simulink model "DTC_section2016b"  (R2016b)
settings: Solver=ode23tb  StartTime=0.0  StopTime=0.4  FixedStep=1e-5  MaxStep=2e-6  RelTol=1e-4  EnableMultiTasking=on
InitFcn:
  | R=1.2;
  | pn=4;
  | Ls=0.0085;
  | phaif=0.175;
libraries: powerlib x5, powerlib_meascontrol x1, simulink x1
settings Model: Creator=miracle  LastModifiedBy=Lei
settings SolverCC: ZeroCrossAlgorithm=Adaptive
settings DataIOCC: SaveFormat=StructureWithTime
settings OptimizationCC: LifeSpan=inf
settings DebuggingCC: SFUnexpectedBacktrackingDiag=warning  SFNoUnconditionalDefaultTransitionDiag=warning  SFExecutionAtInitializationDiag=none
settings HardwareCC: ProdBitPerSizeT=32  ProdBitPerPtrDiffT=32  ProdWordSize=32  ProdHWDeviceType=Specified
settings GRTTargetCC: TargetLangStandard=C89/C90 (ANSI)  GeneratePreprocessorConditionals=Disable all
settings ConfigComp: CovMetricSettings=dw  CovHtmlReporting=on  CovSaveCumulativeToWorkspaceVar=on  CovSaveSingleToWorkspaceVar=on  CovExternalEMLEnable=off
settings SimscapeCC: SimscapeNormalizeSystem=off

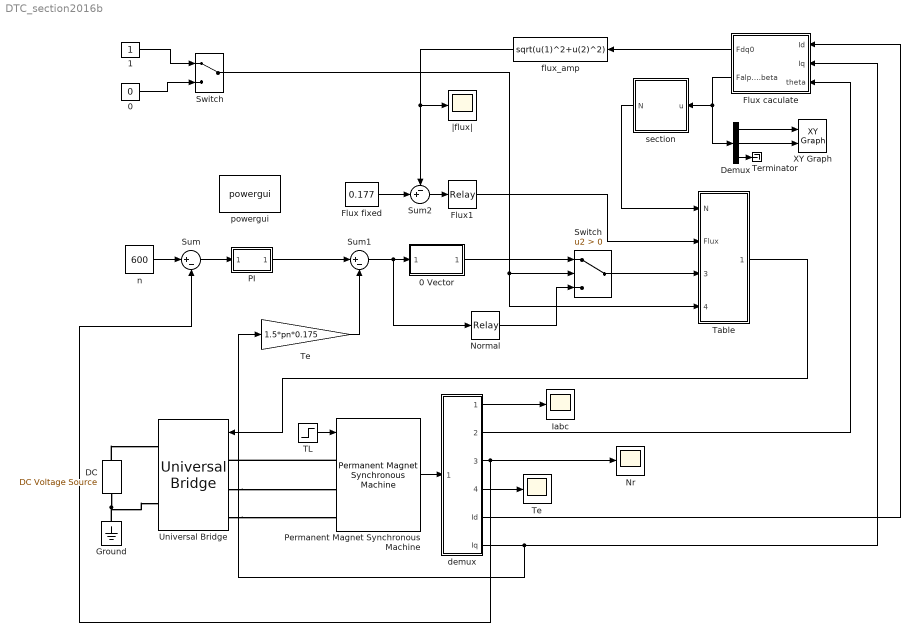
== system DTC_section2016b ==
  " Switch" : ManualSwitch
  0 : Constant  Value=0
  0 Vector : Subsystem
  1 : Constant
  DC : powerlib/Electrical Sources/DC Voltage Source  Amplitude=311  Measurements=None
  Demux : Demux  Outputs=3
  Flux caculate : Subsystem
  Flux fixed : Constant  Value=0.177
  Flux1 : Relay  OnSwitchValue=0.002  OffSwitchValue=-0.002
  Ground : powerlib/Elements/Ground  LConnTagsString=a
  Iabc : Scope
  Normal : Relay  OnSwitchValue=0.15  OffSwitchValue=-0.15
  Nr : Scope
  PI : Subsystem
  Permanent Magnet Synchronous Machine : powerlib/Machines/Permanent Magnet Synchronous Machine  NbPhases=3  FluxDistribution=Sinusoidal  RotorType=Salient-pole  MechanicalLoad=Torque Tm  PresetModel=No  ShowDetailedParameters=on  MeasurementBus=off  Resistance=R  Inductance=8.5e-3  dqInductances=[8.5e-3,8.5e-3]  La=Ls  MachineConstant=Flux linkage established by magnets (V.s)  Flux=phaif  VoltageCst=126.966  TorqueCst=1.05  Flat=120  Mechanical=[0.0008 0.0008 pn 0]  PolePairs=4  InitialConditions=[0,0, 0,0]  InitialConditions5ph=[0 0 0 0 0 0]  TsPowergui=0  TsBlock=-1  RefAngle=Aligned with phase A axis (original Park)
  Sum : Sum  Inputs=|+-
  Sum1 : Sum  Inputs=|+-
  Sum2 : Sum  Inputs=-+|
  Switch : Switch  Criteria=u2 > Threshold
  TL : Step  Time=0.2  After=1.5  SampleTime=0
  Table : Subsystem
  Te : Gain  Gain=1.5*pn*0.175
  "Te " : Scope
  Terminator : Terminator
  Universal Bridge : powerlib/Power Electronics/Universal Bridge  Arms=3  SnubberResistance=1e5  SnubberCapacitance=inf  Device=IGBT / Diodes  Ron=1e-3  Lon=0  ForwardVoltages="[  0  0  ]"  ForwardVoltage=0  GTOparameters=[ 10e-6 , 20e-6 ]  IGBTparameters=[ 1e-6 , 2e-6 ]  Measurements=None  Measurements_2=None  converterType=Rectifier
  XY Graph : simulink/Sinks/XY Graph  xmin=-0.3  xmax=0.3  ymin=-0.3  ymax=0.3  st=-1
  demux : Subsystem
  flux_amp : Fcn  Expr=sqrt(u(1)^2+u(2)^2)
  n : Constant  Value=600
  powergui : powerlib/powergui  Priority=1  SimulationMode=Continuous  SampleTime=50e-6  frequency=60  Iterations=50  frequencyindice=0  Pbase=100e6  ErrMax=1e-4  UnitsV=kV  UnitsW=MW  buscounter=0  FunctionMessages=off  echomessages=off  EnableUseOfTLC=off  CurrentSourceSwitches=on  DisableSnubberDevices=off  DisableRonSwitches=off  DisableVfSwitches=off  DisplayEquations=off  SolverType=Tustin/Backward Euler (TBE)  Interpol=off  ExternalGateDelay=off  methode=off  Ts=10  x0status=blocks  SPID=off  SwTol=0  HookPort=off  RestoreLinks=warning  ResistiveCurrentMeasurement=off  Frange=[0:2:500]  Ylog=off  Xlog=on  ShowGrid=off  save=off  variable=ZData  structure=0  ZoomFFT=off  StartTime=0.0  cycles=1  DisplayStyle=1  fundamental=60  FreqAxis=off  MaxFrequency=1000  frequencyindicesteady=1  RmsSteady=1  display=off
  section : MATLAB Function  TreatAsAtomicUnit=on
  |flux| : Scope
  wires:
  n/1 -> Sum/1
  Sum1/1 -> 0 Vector/1(deltaT), Normal/1
  PI/1(Out1) -> Sum1/1
  TL/1 -> Permanent Magnet Synchronous Machine/1
  Sum2/1 -> Flux1/1
  flux_amp/1 -> Sum2/1, |flux|/1
  section/1(N) -> Table/1(N)
  Sum/1 -> PI/1(In1)
  Permanent Magnet Synchronous Machine/1 -> demux/1(In1)
  demux/5(Id) -> Flux caculate/1(Id)
  demux/1(Iabc) -> Iabc/1
  demux/3(speed) -> Nr/1, Sum/2
  demux/4(Torque) -> "Te "/1
  Flux1/1 -> Table/2(Flux)
  Flux caculate/2(Falpha.beta) -> Demux/1, section/1(u)
  Flux fixed/1 -> Sum2/2
  1/1 -> " Switch"/1
  0/1 -> " Switch"/2
  demux/2(theta) -> Flux caculate/3(theta)
  Table/1(Out1) -> Universal Bridge/1
  " Switch"/1 -> Switch/2, Table/4(Mode)
  Demux/1 -> XY Graph/1
  Demux/2 -> XY Graph/2
  Demux/3 -> Terminator/1
  Flux caculate/1(Fdq0) -> flux_amp/1
  Switch/1 -> Table/3(Torque)
  Normal/1 -> Switch/3
  0 Vector/1(Out1) -> Switch/1
  Te/1 -> Sum1/2
  demux/6(Iq) -> Te/1, Flux caculate/2(Iq)
  connections:
  DC/LConn1 -- Universal Bridge/RConn2 -- Ground/LConn1
  DC/RConn1 -- Universal Bridge/RConn1
  Permanent Magnet Synchronous Machine/LConn1 -- Universal Bridge/LConn1
  Universal Bridge/LConn2 -- Permanent Magnet Synchronous Machine/LConn2
  Universal Bridge/LConn3 -- Permanent Magnet Synchronous Machine/LConn3

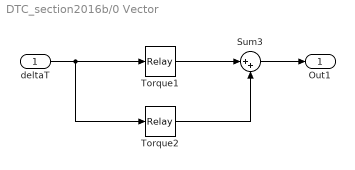
== system DTC_section2016b/0 Vector ==
  deltaT : Inport
  Sum3 : Sum  Inputs=|++
  Torque1 : Relay  OnSwitchValue=0.15  OffSwitchValue=0
  Torque2 : Relay  OnSwitchValue=0  OffSwitchValue=-0.15  OnOutputValue=0  OffOutputValue=-1
  Out1 : Outport
  wires:
  Sum3/1 -> Out1/1
  Torque1/1 -> Sum3/1
  Torque2/1 -> Sum3/2
  deltaT/1 -> Torque2/1, Torque1/1

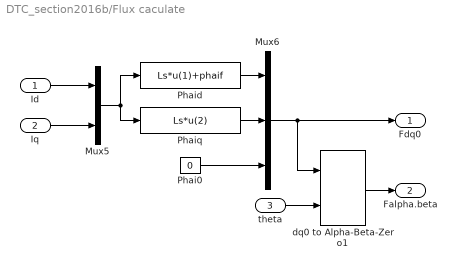
== system DTC_section2016b/Flux caculate ==
  Id : Inport
  Iq : Inport  Port=2
  theta : Inport  Port=3
  Mux5 : Mux  Inputs=2
  Mux6 : Mux  Inputs=3
  Phai0 : Constant  Value=0
  Phaid : Fcn  Expr=Ls*u(1)+phaif
  Phaiq : Fcn  Expr=Ls*u(2)
  dq0 to Alpha-Beta-Zero1 : powerlib_meascontrol/Transformations/dq0 to Alpha-Beta-Zero  Alignment=Aligned with phase A axis
  Fdq0 : Outport
  Falpha.beta : Outport  Port=2
  wires:
  Iq/1 -> Mux5/2
  Id/1 -> Mux5/1
  Phai0/1 -> Mux6/3
  theta/1 -> dq0 to Alpha-Beta-Zero1/2
  Mux6/1 -> Fdq0/1, dq0 to Alpha-Beta-Zero1/1
  dq0 to Alpha-Beta-Zero1/1 -> Falpha.beta/1
  Phaid/1 -> Mux6/1
  Mux5/1 -> Phaiq/1, Phaid/1
  Phaiq/1 -> Mux6/2

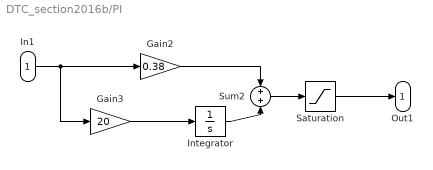
== system DTC_section2016b/PI ==
  In1 : Inport
  Gain2 : Gain  Gain=0.38
  Gain3 : Gain  Gain=20
  Integrator : Integrator  LimitOutput=on  UpperSaturationLimit=5  LowerSaturationLimit=-5
  Saturation : Saturate  UpperLimit=5  LowerLimit=-5
  Sum2 : Sum  Inputs=+|+
  Out1 : Outport
  wires:
  In1/1 -> Gain2/1, Gain3/1
  Gain2/1 -> Sum2/1
  Saturation/1 -> Out1/1
  Gain3/1 -> Integrator/1
  Sum2/1 -> Saturation/1
  Integrator/1 -> Sum2/2

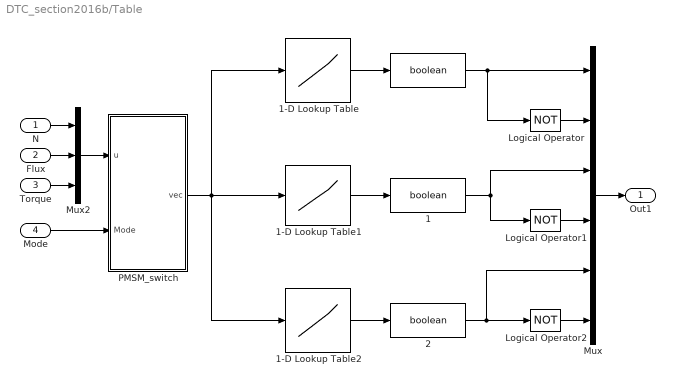
== system DTC_section2016b/Table ==
  N : Inport
  Flux : Inport  Port=2
  Torque : Inport  Port=3
  Mode : Inport  Port=4
  " " : DataTypeConversion  OutDataTypeStr=boolean
  " 1" : DataTypeConversion  OutDataTypeStr=boolean
  " 2" : DataTypeConversion  OutDataTypeStr=boolean
  1-D Lookup Table : Lookup_n-D  NumberOfTableDimensions=1  BreakpointsForDimension1=[1:8]  Table=[0 0 0 1 1 1 1 0]  InternalRulePriority=Speed  RndMeth=Simplest  InputSameDT=on
  1-D Lookup Table1 : Lookup_n-D  NumberOfTableDimensions=1  BreakpointsForDimension1=[1:8]  Table=[0 1 1 0 0 1 1 0]  InternalRulePriority=Speed  RndMeth=Simplest  InputSameDT=on
  1-D Lookup Table2 : Lookup_n-D  NumberOfTableDimensions=1  BreakpointsForDimension1=[1:8]  Table=[1 0 1 0 1 0 1 0]  InternalRulePriority=Speed  RndMeth=Simplest  InputSameDT=on
  Logical Operator : Logic  Operator=NOT  AllPortsSameDT=off  OutDataTypeStr=boolean
  Logical Operator1 : Logic  Operator=NOT  AllPortsSameDT=off  OutDataTypeStr=boolean
  Logical Operator2 : Logic  Operator=NOT  AllPortsSameDT=off  OutDataTypeStr=boolean
  Mux : Mux  Inputs=6
  Mux2 : Mux  Inputs=3
  PMSM_switch : MATLAB Function  TreatAsAtomicUnit=on
  Out1 : Outport
  wires:
  Mux2/1 -> PMSM_switch/1(u)
  PMSM_switch/1(vec) -> 1-D Lookup Table/1, 1-D Lookup Table1/1, 1-D Lookup Table2/1
  1-D Lookup Table/1 -> " "/1
  " "/1 -> Logical Operator/1, Mux/1
  1-D Lookup Table1/1 -> " 1"/1
  " 1"/1 -> Mux/3, Logical Operator1/1
  1-D Lookup Table2/1 -> " 2"/1
  " 2"/1 -> Mux/5, Logical Operator2/1
  Mux/1 -> Out1/1
  Logical Operator/1 -> Mux/2
  Logical Operator1/1 -> Mux/4
  Logical Operator2/1 -> Mux/6
  Torque/1 -> Mux2/3
  Flux/1 -> Mux2/2
  N/1 -> Mux2/1
  Mode/1 -> PMSM_switch/2(Mode)

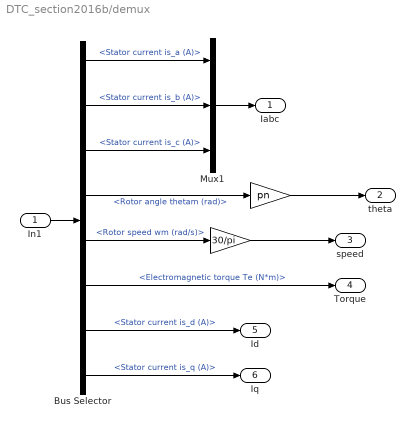
== system DTC_section2016b/demux ==
  In1 : Inport
  "  " : Gain  Gain=30/pi
  "   " : Gain  Gain=pn
  Bus Selector : BusSelector  OutputSignals=Stator current is_a (A),Stator current is_b (A),Stator current is_c (A),Rotor angle thetam (rad),Rotor speed wm (rad/s),Electromagnetic torque Te (N*m),Stator current is_d (A),Stator current is_q (A)
  Mux1 : Mux  Inputs=3
  Iabc : Outport
  theta : Outport  Port=2
  speed : Outport  Port=3
  Torque : Outport  Port=4
  Id : Outport  Port=5
  Iq : Outport  Port=6
  wires:
  In1/1 -> Bus Selector/1
  Bus Selector/1 -> Mux1/1  "<Stator current is_a (A)>"
  Bus Selector/2 -> Mux1/2  "<Stator current is_b (A)>"
  Bus Selector/3 -> Mux1/3  "<Stator current is_c (A)>"
  Bus Selector/6 -> Torque/1  "<Electromagnetic torque Te (N*m)>"
  Bus Selector/5 -> "  "/1  "<Rotor speed wm (rad/s)>"
  "  "/1 -> speed/1
  Mux1/1 -> Iabc/1
  Bus Selector/4 -> "   "/1  "<Rotor angle thetam (rad)>"
  "   "/1 -> theta/1
  Bus Selector/7 -> Id/1  "<Stator current is_d (A)>"
  Bus Selector/8 -> Iq/1  "<Stator current is_q (A)>"

== matlab function DTC_section2016b/Table/PMSM_switch ==
  data: u input; vec output; Mode input
function vec = PMSM_switch(u,Mode)
u(1)=round(u(1));   %扇区
V_Table0 = [ 1 5 4 6 2 3 ; 2 3 1 5 4 6 ; 5 4 6 2 3 1 ; 6 2 3 1 5 4];    %无零矢量模式下的开关表，表4-2
V_Table1 = [ 1 5 4 6 2 3 ; 8 7 8 7 8 7 ; 2 3 1 5 4 6 ; 5 4 6 2 3 1 ; 7 8 7 8 7 8 ;6 2 3 1 5 4]; %含零矢量模式下的开关表，表4-3

vec = 1;	%默认选择U1矢量
if Mode==0  %无零矢量模式
    x=2*u(2)+ u(3)+1;
    vec = V_Table0(x,u(1));
    return;
end

if Mode==1  %含零矢量模式
    x=3*u(2)+ u(3)+2;
    vec = V_Table1(x,u(1));
    return;
end

== matlab function DTC_section2016b/section ==
  data: u input; N output size=1
function N = section(u)
a1=u(1);    %磁链在U4矢量方向上的投影
b1=u(1)*(-0.5)+(sqrt(3)/2)*u(2);%磁链在U2矢量方向上的投影
c1=u(1)*(-0.5)-(sqrt(3)/2)*u(2);%磁链在U1矢量方向上的投影

if a1>0
    a=0;
else
    a=1;
end

if b1>0
    b=0;
else
    b=1;
end

if c1>0
    c=0;
else
    c=1;
end

N1 = 4*a+2*b+c; %扇区计算中间量
switch N1       %将扇区变换成图4-4所示的划分方式
    case 1
        N=2;
    case 2
        N=6;
    case 3
        N=1;
    case 4
        N=4;
    case 5
        N=3;
    case 6
        N=5;
    otherwise
        N=1;    %默认在第一扇区
end
